simulink model "prestoAJ_a448_Reentry_vA_Sim"  (R2024a)
settings: Solver=VariableStepAuto  StartTime=0.0  StopTime=tspan  RelTol=1e-9
values from neighbouring files (symbols this model uses):
  Cd = 0.02723    [prestoAJ_a448_Reentry.m]
  CL = 0.11059    [prestoAJ_a448_Reentry.m]
  H = 7100    [prestoAJ_a448_Reentry.m]
  m_reentry = m_dry + m_prop*.05    (= 90200)    [prestoAJ_a448_Reentry.m]
  mu = 3.986004418e14    (= 398600441800000)    [prestoAJ_a448_Reentry.m]
  OmegaE = 7.2921159e-5    (= 7.2921159e-05)    [prestoAJ_a448_Reentry.m]
  rE = 6378000    [prestoAJ_a448_Reentry.m]
  rho0 = 1.225    [prestoAJ_a448_Reentry.m]
  S = 138    [prestoAJ_a448_Reentry.m]
  x0 = 0    [main_simulation.m]    (also in prestoAJ_a448_Reentry.m = [r0;lon0;lat0;v0;y0;psi0])
undefined symbols (not defined in the file or in its folder): r_ECI_0, v_ECI_0
libraries: simulink x1
settings Model: Creator=prest  LastModifiedBy=prest

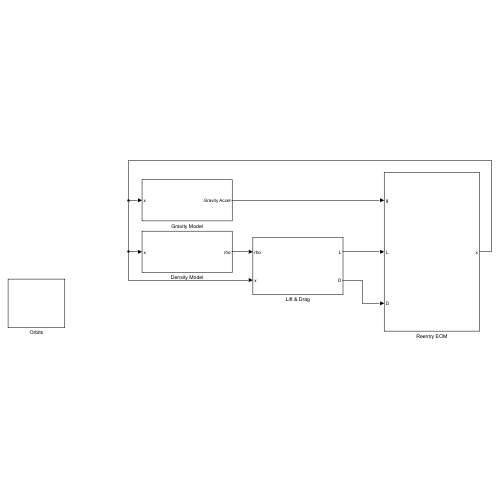
[thumbnail: Simulink's stored preview of the top-level diagram]
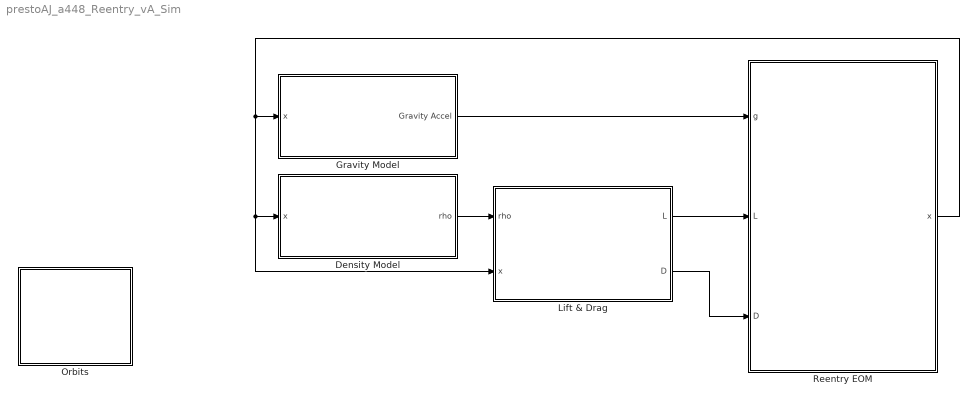
== system prestoAJ_a448_Reentry_vA_Sim ==
  Density Model : Subsystem
  Gravity Model : Subsystem
  Lift & Drag : Subsystem
  Orbits : Subsystem
  Reentry EOM : Subsystem
  wires:
  Reentry EOM/1(x) -> Density Model/1(x), Lift & Drag/2(x), Gravity Model/1(x)
  Density Model/1(rho) -> Lift & Drag/1(rho)
  Gravity Model/1(Gravity Accel) -> Reentry EOM/1(g)
  Lift & Drag/1(L) -> Reentry EOM/2(L)
  Lift & Drag/2(D) -> Reentry EOM/3(D)

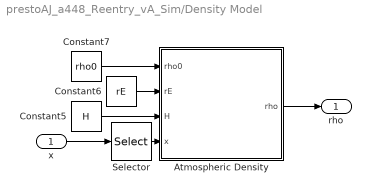
== system prestoAJ_a448_Reentry_vA_Sim/Density Model ==
  x : Inport
  Atmospheric Density : MATLAB Function  TreatAsAtomicUnit=on
  Constant5 : Constant  Value=H  VectorParams1D=off
  Constant6 : Constant  Value=rE  VectorParams1D=off
  Constant7 : Constant  Value=rho0  VectorParams1D=off
  Selector : Selector  InputPortWidth=6  IndexOptions=Index vector (dialog)  Indices=1  OutputSizes=1
  rho : Outport
  wires:
  Constant5/1 -> Atmospheric Density/3(H)
  Constant6/1 -> Atmospheric Density/2(rE)
  Constant7/1 -> Atmospheric Density/1(rho0)
  Atmospheric Density/1(rho) -> rho/1
  Selector/1 -> Atmospheric Density/4(x)
  x/1 -> Selector/1

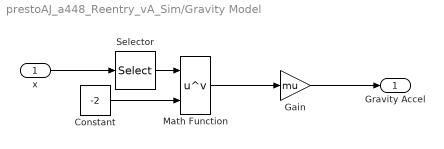
== system prestoAJ_a448_Reentry_vA_Sim/Gravity Model ==
  x : Inport
  Constant : Constant  Value=-2  VectorParams1D=off
  Gain : Gain  Gain=mu
  Math Function : Math  Operator=pow  SignedPower=on
  Selector : Selector  InputPortWidth=6  IndexOptions=Index vector (dialog)  Indices=1  OutputSizes=1
  Gravity Accel : Outport
  wires:
  Gain/1 -> Gravity Accel/1
  Math Function/1 -> Gain/1
  Constant/1 -> Math Function/2
  x/1 -> Selector/1
  Selector/1 -> Math Function/1

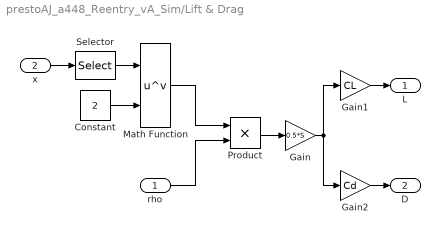
== system prestoAJ_a448_Reentry_vA_Sim/Lift & Drag ==
  rho : Inport
  x : Inport  Port=2
  Constant : Constant  Value=2  VectorParams1D=off
  Gain : Gain  Gain=0.5*S
  Gain1 : Gain  Gain=CL
  Gain2 : Gain  Gain=Cd
  Math Function : Math  Operator=pow  SignedPower=on
  Product : Product
  Selector : Selector  InputPortWidth=6  IndexOptions=Index vector (dialog)  Indices=4  OutputSizes=1
  L : Outport
  D : Outport  Port=2
  wires:
  x/1 -> Selector/1
  Selector/1 -> Math Function/1
  Constant/1 -> Math Function/2
  Math Function/1 -> Product/1
  rho/1 -> Product/2
  Product/1 -> Gain/1
  Gain1/1 -> L/1
  Gain/1 -> Gain2/1, Gain1/1
  Gain2/1 -> D/1

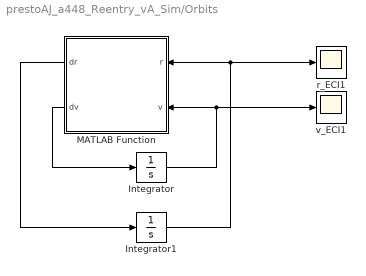
== system prestoAJ_a448_Reentry_vA_Sim/Orbits ==
  Integrator : Integrator  InitialCondition=v_ECI_0
  Integrator1 : Integrator  InitialCondition=r_ECI_0
  MATLAB Function : MATLAB Function  TreatAsAtomicUnit=on
  r_ECI1 : Scope
  v_ECI1 : Scope
  wires:
  Integrator/1 -> v_ECI1/1, MATLAB Function/2(v)
  Integrator1/1 -> r_ECI1/1, MATLAB Function/1(r)
  MATLAB Function/1(dr) -> Integrator1/1
  MATLAB Function/2(dv) -> Integrator/1

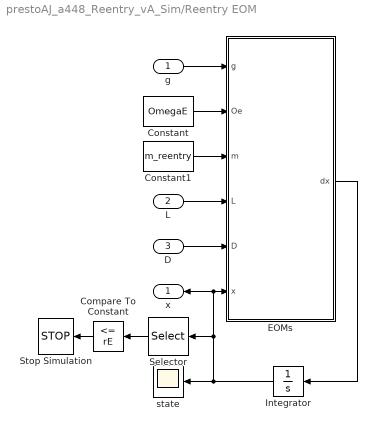
== system prestoAJ_a448_Reentry_vA_Sim/Reentry EOM ==
  g : Inport
  L : Inport  Port=2
  D : Inport  Port=3
  Compare To Constant : simulink/Logic and Bit Operations/Compare To Constant  relop=<=  const=rE  OutDataTypeStr=boolean
  Constant : Constant  Value=OmegaE  VectorParams1D=off
  Constant1 : Constant  Value=m_reentry  VectorParams1D=off
  EOMs : MATLAB Function  TreatAsAtomicUnit=on
  Integrator : Integrator  InitialCondition=x0
  Selector : Selector  InputPortWidth=6  IndexOptions=Index vector (dialog)  Indices=1  OutputSizes=1
  Stop Simulation : Stop
  state : Scope
  x : Outport
  wires:
  EOMs/1(dx) -> Integrator/1
  Constant/1 -> EOMs/2(Oe)
  Integrator/1 -> state/1, x/1, EOMs/6(x), Selector/1
  Constant1/1 -> EOMs/3(m)
  g/1 -> EOMs/1(g)
  D/1 -> EOMs/5(D)
  L/1 -> EOMs/4(L)
  Compare To Constant/1 -> Stop Simulation/1
  Selector/1 -> Compare To Constant/1

== matlab function prestoAJ_a448_Reentry_vA_Sim/Density Model/Atmospheric Density ==
  data: rho0 input; rE input; H input; x input; rho output
function rho = Density(rho0, rE, H, x)

rho = rho0*exp(-(x(1)-rE)/H); % [kg/m^3] Current Atmospheric Density

== matlab function prestoAJ_a448_Reentry_vA_Sim/Reentry EOM/EOMs ==
  data: g input; Oe input; m input; L input; D input; dx output; x input
function dx  = ReentryEOM(g, Oe, m, L, D, x)

% Calculate/Declare Constants
sig = 0; % [rad] Bank angle (Might change location later)

% Calculate derivative of state vector
dx = zeros(6,1);
dx(1) = x(4)*sin(x(5));
dx(2) = x(4)*cos(x(5))*sin(x(6))/x(1)/cos(x(3));
dx(3) = x(4)*cos(x(5))*cos(x(6))/x(1);
dx(4) = -D/m - g*sin(x(5)) + Oe^2*x(1)*cos(x(3))*(sin(x(5))*cos(x(3))-cos(x(5))*sin(x(3))*cos(x(6)));
dx(5) = (L*cos(sig)/m - g*cos(x(5)) + x(4)^2*cos(x(5))/x(1) + 2*Oe*x(4)*cos(x(3))*sin(x(6)) + Oe^2*x(1)*cos(x(3))*(cos(x(5))*cos(x(3)) + sin(x(5))*cos(x(6))*sin(x(3))))/x(4);
dx(6) = (L*sin(sig)/m/cos(x(5)) + x(4)^2*cos(x(5))*sin(x(6))*tan(x(3))/x(1) -  2*Oe*x(4)*(tan(x(5))*cos(x(6))*cos(x(3)) - sin(x(3))) + Oe^2*x(1)*sin(x(6))*sin(x(3))*cos(x(3))/cos(x(5)))/x(4);

== matlab function prestoAJ_a448_Reentry_vA_Sim/Orbits/MATLAB Function ==
  data: r input; dr output; v input; dv output
function [dr,dv] = orbitalDynamics(r, v)
    mu = 398600;
    rnorm = norm(r);
    a = -mu.*r(:)./(rnorm^3);
    
    dr = v(:);
    dv = a(:);
